simulink model "main"  (R2021a)
settings: Solver=VariableStepAuto  StartTime=0.0  StopTime=0.05  RelTol=1e-3
libraries: visionsources x4, pid_lib x1
settings Model: Creator=win10  LastModifiedBy=win10

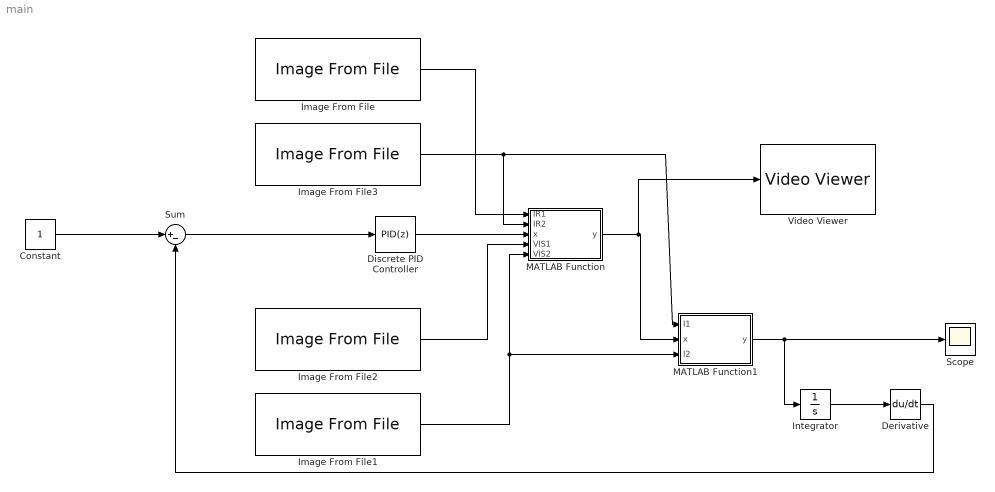
== system main ==
  Constant : Constant
  Derivative : Derivative
  Discrete PID Controller : pid_lib/PID Controller  Controller=PID  Form=Parallel  TimeDomain=Discrete-time  UseExternalTs=off  SampleTime=-1  IntegratorMethod=Forward Euler  FilterMethod=Forward Euler  ControllerParametersSource=internal  P=0.6  I=0.1  D=0  UseFilter=on  N=100  TunerSelectOption=Transfer Function Based (PID Tuner App)  InitialConditionSource=internal  InitialConditionForIntegrator=0  InitialConditionForFilter=0  DifferentiatorICPrevScaledInput=0  ExternalReset=none  TrackingMode=off  Kt=1  LimitOutput=off  SatLimitsSource=internal  UpperSaturationLimit=inf  LowerSaturationLimit=-inf  LinearizeAsGain=off  AntiWindupMode=none  Kb=1  POutMin=[]  POutMax=[]  IOutMin=[]  IOutMax=[]  DOutMin=[]  DOutMax=[]  NOutMin=[]  NOutMax=[]  SumOutMin=[]  SumOutMax=[]  SaturationOutMin=[]  SaturationOutMax=[]  PParamMin=[]  PParamMax=[]  IParamMin=[]  IParamMax=[]  DParamMin=[]  DParamMax=[]  NParamMin=[]  NParamMax=[]  KbParamMin=[]  KbParamMax=[]  KtParamMin=[]  KtParamMax=[]  KbOutMin=[]  KbOutMax=[]  KtOutMin=[]  KtOutMax=[]  IntegratorOutMin=[]  IntegratorOutMax=[]  FilterOutMin=[]  FilterOutMax=[]  SumI1OutMin=[]  SumI1OutMax=[]  SumI2OutMin=[]  SumI2OutMax=[]  SumI3OutMin=[]  SumI3OutMax=[]  SumI4OutMin=[]  SumI4OutMax=[]  SumDOutMin=[]  SumDOutMax=[]  DifferentiatorOutMin=[]  DifferentiatorOutMax=[]  FilterDiffOutCoefMin=[]  FilterDiffOutCoefMax=[]  ReciprocalOutMin=[]  ReciprocalOutMax=[]  SumDenOutMin=[]  SumDenOutMax=[]  SumNumOutMin=[]  SumNumOutMax=[]  DivideOutMin=[]  DivideOutMax=[]  UdiffTsProdOutMin=[]  UdiffTsProdOutMax=[]  NTsProdOutMin=[]  NTsProdOutMax=[]  UintegralTsProdOutMin=[]  UintegralTsProdOutMax=[]  UngainTsProdOutMin=[]  UngainTsProdOutMax=[]  IntegratorContinuousStateAttributes=''  IntegratorStateMustResolveToSignalObject=off  IntegratorRTWStateStorageClass=Auto  FilterContinuousStateAttributes=''  FilterStateMustResolveToSignalObject=off  FilterRTWStateStorageClass=Auto  ParallelPVariant=InternalParameters  IdealPVariant=Disabled  IVariant=InternalParameters  DVariant=InternalParameters  IntegratorVariant=Discrete  SatVariant=Disabled  AWVariant=Passthrough  PCopyVariant=Disabled  TRVariant=Disabled  FdbkBlocksVariant=Forward  IdealPFdbkVariant=Disabled  SatFdbkVariant=Disabled  DerivativeFilterVariant=ForwardEulerFilter  NVariant=InternalParameters  NCopyVariant=Disabled  FilterICVariant=InternalICsFilter  IntegratorICVariant=InternalICs  ExternalResetVariant=Disabled  TRSumVariant=Passthrough  SumFdbkVariant=Disabled  SumVariant=Sum_PID  TsampFilterVariant=InternalTs  TsampNgainVariant=Passthrough  TsampIntegralVariant=Passthrough  ExternalSaturationOutDataTypeStr=Inherit: Same as second input
  Image From File : visionsources/Image From File  Tag=vipblks_nd  FileName=E:\ShiYan\2.1\samples\49IR.bmp  Ts=inf  imagePorts=One multidimensional signal  OutPortLabels=R|G|B  ImageDataType=Inherit from input image  sdImageDataType=uint(8)  Signed=on  WordLength=16  FractionLengthMode=User-defined  FractionLength=15
  Image From File1 : visionsources/Image From File  Tag=vipblks_nd  FileName=E:\ShiYan\2.1\samples\50VIS.bmp  Ts=inf  imagePorts=One multidimensional signal  OutPortLabels=R|G|B  ImageDataType=Inherit from input image  sdImageDataType=uint(8)  Signed=on  WordLength=16  FractionLengthMode=User-defined  FractionLength=15
  Image From File2 : visionsources/Image From File  Tag=vipblks_nd  FileName=E:\ShiYan\2.1\samples\49VIS.bmp  Ts=inf  imagePorts=One multidimensional signal  OutPortLabels=R|G|B  ImageDataType=Inherit from input image  sdImageDataType=uint(8)  Signed=on  WordLength=16  FractionLengthMode=User-defined  FractionLength=15
  Image From File3 : visionsources/Image From File  Tag=vipblks_nd  FileName=E:\ShiYan\2.1\samples\50IR.bmp  Ts=inf  imagePorts=One multidimensional signal  OutPortLabels=R|G|B  ImageDataType=Inherit from input image  sdImageDataType=uint(8)  Signed=on  WordLength=16  FractionLengthMode=User-defined  FractionLength=15
  Integrator : Integrator
  MATLAB Function : MATLAB Function  TreatAsAtomicUnit=on
  MATLAB Function1 : MATLAB Function  TreatAsAtomicUnit=on
  Scope : Scope
  Sum : Sum  Inputs=|+-
  Video Viewer : VideoViewer  FigPos=[1383 541 357 315]
  wires:
  Sum/1 -> Discrete PID Controller/1
  Discrete PID Controller/1 -> MATLAB Function/3(x)
  MATLAB Function/1(y) -> Video Viewer/1, MATLAB Function1/2(x)
  MATLAB Function1/1(y) -> Integrator/1, Scope/1
  Image From File/1 -> MATLAB Function/1(IR1)
  Image From File3/1 -> MATLAB Function/2(IR2), MATLAB Function1/1(I1)
  Image From File2/1 -> MATLAB Function/4(VIS1)
  Image From File1/1 -> MATLAB Function1/3(I2), MATLAB Function/5(VIS2)
  Integrator/1 -> Derivative/1
  Derivative/1 -> Sum/2
  Constant/1 -> Sum/1

== matlab function main/MATLAB Function1 ==
  data: I1 input; y output; x input; I2 input
function y = Qabf1(I1,x,I2)
A=(I1);
B=(I2);
F=(x);
 
if size(A,3)==3
    ppA=rgb2gray(A);
else
    ppA=A;
end
if size(B,3)==3
    ppB=rgb2gray(B);
else
    ppB=B;
end
if size(F,3)==3
    ppF=rgb2gray(F);
else
    ppF=F;
end
% 尺寸标准化
[M,N]=size(ppA);
if mod(M,2)==1 && mod(N,2)==1
%     pA=zeros(M-1,N-1);
%     pB=zeros(M-1,N-1);
%     pF=zeros(M-1,N-1);
    pA=imresize(ppA,[M-1,N-1]);
    pB=imresize(ppB,[M-1,N-1]);
    pF=imresize(ppF,[M-1,N-1]);
end
if mod(M,2)==1 && mod(N,2)==0
%     pA=zeros(M-1,N);
%     pB=zeros(M-1,N);
%     pF=zeros(M-1,N);
    pA=imresize(ppA,[M-1,N]);
    pB=imresize(ppB,[M-1,N]);
    pF=imresize(ppF,[M-1,N]);
end
if mod(M,2)==0 && mod(N,2)==1
%     pA=zeros(M,N-1);
%     pB=zeros(M,N-1);
%     pF=zeros(M,N-1);
    pA=imresize(ppA,[M,N-1]);
    pB=imresize(ppB,[M,N-1]);
    pF=imresize(ppF,[M,N-1]);
end
if mod(M,2)==0 && mod(N,2)==0
pA=ppA;
pB=ppB;
pF=ppF;
end

pA = im2double(pA);
pB = im2double(pB);
pF = im2double(pF);
   L=1; Tg=0.9994;kg=-15;Dg=0.5;Ta=0.9879;ka=-22;Da=0.8;       
 
h1=[1 2 1;0 0 0;-1 -2 -1]; h2=[0 1 2;-1 0 1;-2 -1 0]; h3=[-1 0 1;-2 0 2;-1 0 1];
SAx = conv2(pA,h3,'same'); SAy = conv2(pA,h1,'same');
gA = sqrt(SAx.^2 + SAy.^2); 
[M,N] = size(SAx); aA = zeros(M,N);
for i=1:M
    for j=1:N
        if ( SAx(i,j) == 0 ) aA(i,j) = pi/2;
        else
            aA(i,j) = atan(SAy(i,j)/SAx(i,j));
        end
    end
end
 
SBx = conv2(pB,h3,'same'); SBy = conv2(pB,h1,'same');
gB = sqrt(SBx.^2 + SBy.^2); 
[M,N] = size(SBx); aB = zeros(M,N);
for i=1:M
    for j=1:N
        if ( SBx(i,j) == 0 ) aB(i,j) = pi/2;
        else
            aB(i,j) = atan(SBy(i,j)/SBx(i,j));
        end
    end
end
 
SFx = conv2(pF,h3,'same'); SFy = conv2(pF,h1,'same');
gF = sqrt(SFx.^2 + SFy.^2); 
[M,N] = size(SAx); aF = zeros(M,N);
for i=1:M
    for j=1:N
        if ( SFx(i,j) == 0 ) aF(i,j) = pi/2;
        else
            aF(i,j) = atan(SFy(i,j)/SFx(i,j));
        end
    end
end
 
% the relative strength and orientation value of GAF,GBF and AAF,ABF;
GAF = zeros(M,N); AAF = zeros(M,N); QgAF = zeros(M,N); QaAF = zeros(M,N); QAF = zeros(M,N);
for i=1:M
    for j=1:N
        
        if ( gA(i,j) > gF(i,j))  GAF(i,j) = gF(i,j)/gA(i,j);
        else
            if ( gA(i,j) == gF(i,j) )  GAF(i,j) = gF(i,j);
            else
                GAF(i,j) = gA(i,j) / gF(i,j);
            end
        end 
        AAF(i,j) = 1 - abs(aA(i,j)-aF(i,j))/(pi/2);
        
        QgAF(i,j) = Tg / (1 + exp(kg*( GAF(i,j) - Dg )));
        QaAF(i,j) = Ta / (1 + exp(ka*( AAF(i,j) - Da )));
        
        QAF(i,j) = QgAF(i,j) * QaAF(i,j);
    end
end
 
GBF2 = zeros(M,N);GBF1 = zeros(M,N);GBF = zeros(M,N); ABF = zeros(M,N); QgBF = zeros(M,N); QaBF = zeros(M,N); QBF = zeros(M,N);
for i=1:M
    for j=1:N
        
        if ( gB(i,j) > gF(i,j))  GBF(i,j) = gF(i,j)/gB(i,j);
        else
            if ( gB(i,j) == gF(i,j) )  GBF(i,j) = gF(i,j);
            else
                GBF(i,j) = gB(i,j) / gF(i,j);
            end
        end 
        ABF(i,j) = 1 - abs(aB(i,j)-aF(i,j))/(pi/2);
        
        QgBF(i,j) = Tg / (1 + exp(kg*( GBF(i,j) - Dg )));
        QaBF(i,j) = Ta / (1 + exp(ka*( ABF(i,j) - Da )));
        
        QBF(i,j) = QgBF(i,j) * QaBF(i,j);
    end
end
 
for i=1:M
    for j=1:N
        if ( gB(i,j) > gF(i,j))||(gA(i,j) > gF(i,j))
            GBF1(i,j)=1;
        else
            GBF1(i,j)=0;
        end 
    end
end
 
for i=1:M
    for j=1:N
        if gF(i,j)>(gA(i,j)&gF(i,j))
            GBF2(i,j)=2-QAF(i,j)-QBF(i,j);
        else
            GBF2(i,j)=0;
        end 
    end
end
 
 
deno = sum(sum( gA + gB ));
nume = sum(sum( QAF.*gA + QBF.*gB ));
y=(nume / deno);

end

== matlab function main/MATLAB Function ==
  data: IR1 input; y output; IR2 input; x input; VIS1 input; VIS2 input
function y=fcn(IR1,IR2,x,VIS1,VIS2)
% 图像灰度化
if size(IR1,3)>1
    IR_1=rgb2gray(IR1);
else
    IR_1=IR1;
end
if size(IR2,3)>1
    IR_2=rgb2gray(IR2);
else
    IR_2=IR2;
end
if size(VIS1,3)>1
    VIS_1=rgb2gray(VIS1);
else
    VIS_1=VIS1;
end
if size(VIS2,3)>1
    VIS_2=rgb2gray(VIS2);
else
    VIS_2=VIS2;
end
% 图像大小标准化
[row1,col1]=size(IR_1);
if mod(row1,2)==1
    row1=row1-1;
end
if mod(col1,2)==1
    col1=col1-1;
end
ir_1=zeros(row1,col1);
ir_1=imresize(IR_1,[row1,col1]);

[row2,col2]=size(IR_2);
if mod(row2,2)==1
    row2=row2-1;
end
if mod(col2,2)==1
    col2=col2-1;
end
ir_2=zeros(row2,col2);
ir_2=imresize(IR_2,[row2,col2]);

[row3,col3]=size(VIS_1);
if mod(row3,2)==1
    row3=row3-1;
end
if mod(col3,2)==1
    col3=col3-1;
end
vis_1=zeros(row3,col3);
vis_1=imresize(VIS_1,[row3,col3]);

[row4,col4]=size(VIS_2);
if mod(row4,2)==1
    row4=row4-1;
end
if mod(col4,2)==1
    col4=col4-1;
end
vis_2=zeros(row4,col4);
vis_2=imresize(VIS_2,[row4,col4]);

M=row1;
N=col1;

% 提取局部差分特征
[A1,A2,A3,A4,A22,A33,A44] = Fenk(ir_1,M,N);
[B1,B2,B3,B4,B22,B33,B44] = Fenk(ir_2,M,N);
[C1,C2,C3,C4,C22,C33,C44] = Fenk(vis_1,M,N);
[D1,D2,D3,D4,D22,D33,D44] = Fenk(vis_2,M,N);

% 提取关联细节特征
P2=Fea(A2,B2,M,N);
P3=Fea(A3,B3,M,N);
P4=Fea(A4,B4,M,N);
P22=Fea(A22,B22,M,N);
P33=Fea(A33,B33,M,N);
P44=Fea(A44,B44,M,N);
Q2=Fea(C2,D2,M,N);
Q3=Fea(C3,D3,M,N);
Q4=Fea(C4,D4,M,N);
Q22=Fea(C22,D22,M,N);
Q33=Fea(C33,D33,M,N);
Q44=Fea(C44,D44,M,N);

% 红外显著性目标提取
Ig=double(ir_2);
I1=log(Ig+1);%取对数
FI=fft2(I1);%傅里叶变换
n1=floor(M/2);
n2=floor(N/2);
D=zeros(M,N);
H=zeros(M,N);
% k=-200;
for i=1:M
   for j=1:N      
       D(i,j)=((i-n1).^2+(j-n2).^2);
% H(i,j)=(rH-rL).*(exp(c*(-D(i,j)./(d0^2))))+rL; %高斯同态滤波              
       H(i,j)=85./(1+exp(1./(D(i,j))));
  end
end
I2=ifft2(H.*FI);
I33=real(exp(I2));
I33=I33./(10^144);
I3=zeros(M,N);
ma=max(I33(:));
mi=min(I33(:));
for i=1:M
    for j=1:N
        I3(i,j)=round(255.*(I33(i,j)-mi)./(ma-mi));
    end
end
avg=mean(mean(I3(:)));
Ig(I3(:)<avg)=0;
% 计算边缘强度
E_ir=metricsEdge_intensity(double(ir_2));
E_vis=metricsEdge_intensity(double(vis_2));
We=0.5.*E_ir./(E_ir+E_vis);
% 细节层融合
FPQ2=Fuse_d(P2,Q2,We);
PPQ3=Fuse_d(P3,Q3,We);
FPQ4=Fuse_d(P4,Q4,We);
FPQ22=Fuse_d(P22,Q22,We);
FPQ33=Fuse_d(P33,Q33,We);
FPQ44=Fuse_d(P44,Q44,We);

% 基层融合
SD_B=SD(double(ir_2));
SD_D=SD(double(vis_2));
% Eta=exp(((SD_B-SD_D)./SD_D).^(abs(SD_B-SD_D)./(SD_B-SD_D)));

Eta=exp(((SD_B-SD_D)./(SD_B+SD_D)).^(abs(SD_B-SD_D)./(SD_B-SD_D)));

FBD1=B1.*(x+0.5.*Eta)+D1.*(x+0.5);
F=Inverse_Fenk(FBD1,FPQ2,PPQ3,FPQ4,FPQ22,FPQ33,FPQ44,M,N);
y=uint8(F+Ig);

end
